simulink model "HLF_SystemArchitecture"  (R2024a)
settings: Solver=VariableStepAuto  StartTime=0.0  StopTime=10.0  RelTol=1e-3
undefined symbols (not defined in the file): Deceleration, LIN_Acceleration
settings Model: DataDictionary=DD_HLF_DataTypes.sldd  Creator=The MathWorks, Inc.  LastModifiedBy=The MathWorks, Inc.
settings SolverCC: AlgebraicLoopSolver=TrustRegion  MaxZcPerStep=1
settings DebuggingCC: UnconnectedInputMsg=warning  UnconnectedOutputMsg=warning  UnconnectedLineMsg=warning
settings ModelReferenceCC: EnableRefExpFcnMdlSchedulingChecks=on
settings RTWCC: GPUComputeCapability=3.5  DLArmComputeVersion=19.05

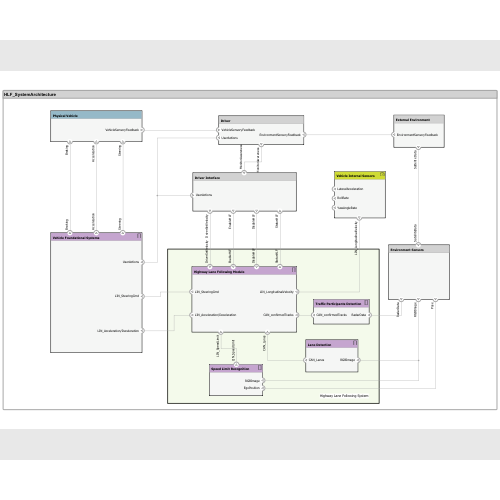
[thumbnail: Simulink's stored preview of the top-level diagram]
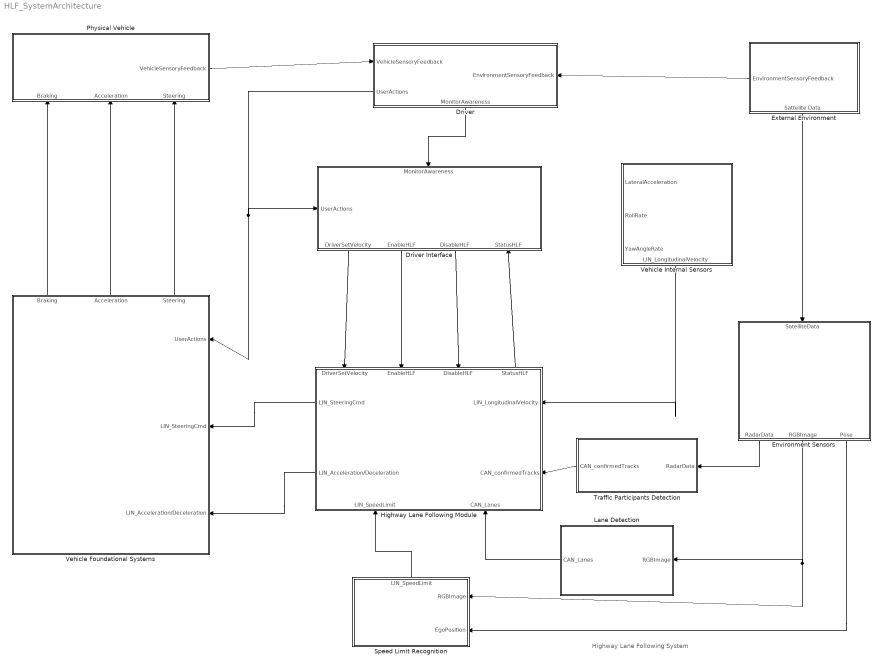
== system HLF_SystemArchitecture ==
  note: Highway Lane Following System
  Driver : Subsystem
      settings: PortSchema="{\"entries\":[{\"content\":{\"headerSize\":26,\"margin\":15,\"minimumSpacing\":25,\"sides\":[{\"content\":{\"connectorIds\":[\"In1\",\"Out2\"]},\"type\":\"ConnectorPlacement.EquallySpacedRectSide\",\"uuid\":\"57d9105b-5891-4b67-8053-94876359dbfc\"},{\"content\":{\"connectorIds\":[\"In2\"],\"side\":\"RIGHT\"},\"type\":\"ConnectorPlacement.EquallySpacedRectSide\",\"uuid\":\"3fd4430d-d88a-4c36-b7db-738c17ba6bd1\"},{\"content\":{\"connectorIds\":[],\"side\":\"TOP\"},\"type\":\"ConnectorPlacement.EquallySpacedRectSide\",\"uuid\":\"61a8faa4-d042-4724-a03b-b771d37b6fdb\"},{\"content\":{\"connectorIds\":[\"Out1\"],\"side\":\"BOTTOM\"},\"type\":\"ConnectorPlacement.EquallySpacedRectSide\",\"uuid\":\"67674867-d4fb-4781-a637-daf086112980\"},{\"content\":{\"connectorIds\":[],\"side\":\"HIDDEN\"},\"type\":\"ConnectorPlacement.EquallySpacedRectSide\",\"uuid\":\"dc3c6b25-4da2-48ee-a238-2c1d12fb30ea\"}]},\"type\":\"ConnectorPlacement.EquallySpacedConnector\",\"uuid\":\"fbcd43a8-976e-4463-97d1-0d40c2a22b40\"}],\"packageUris\":[\"http://schema.mathworks.com/mf0/Connector/R2020b\"],\"version\":\"1.0\"}"
  Driver Interface : Subsystem
      settings: PortSchema="{\"entries\":[{\"content\":{\"headerSize\":26,\"margin\":15,\"minimumSpacing\":25,\"sides\":[{\"content\":{\"connectorIds\":[\"In3\"]},\"type\":\"ConnectorPlacement.EquallySpacedRectSide\",\"uuid\":\"b5c560bf-b1de-4f7d-bfcc-f34083c77ac8\"},{\"content\":{\"connectorIds\":[],\"side\":\"RIGHT\"},\"type\":\"ConnectorPlacement.EquallySpacedRectSide\",\"uuid\":\"ae8c8d4f-55e3-4192-b0d3-7950d45edb35\"},{\"content\":{\"connectorIds\":[\"In2\"],\"side\":\"TOP\"},\"type\":\"ConnectorPlacement.EquallySpacedRectSide\",\"uuid\":\"be988242-c8a1-4b97-b048-993c7975a175\"},{\"content\":{\"connectorIds\":[\"Out1\",\"Out2\",\"Out3\",\"In1\"],\"side\":\"BOTTOM\"},\"type\":\"ConnectorPlacement.EquallySpacedRectSide\",\"uuid\":\"b880dce2-1370-4b6b-af53-719174202621\"},{\"content\":{\"connectorIds\":[],\"side\":\"HIDDEN\"},\"type\":\"ConnectorPlacement.EquallySpacedRectSide\",\"uuid\":\"95e462f2-ec2c-4474-9ace-7d27c2e08c82\"}]},\"type\":\"ConnectorPlacement.EquallySpacedConnector\",\"uuid\":\"71deff37-1671-43b5-b896-1963241a26e4\"}],\"packageUris\":[\"http://schema.mathworks.com/mf0/Connector/R2020b\"],\"version\":\"1.0\"}"
  Environment Sensors : Subsystem
      settings: PortSchema="{\"entries\":[{\"content\":{\"headerSize\":26,\"margin\":15,\"minimumSpacing\":25,\"sides\":[{\"content\":{\"connectorIds\":[]},\"type\":\"ConnectorPlacement.EquallySpacedRectSide\",\"uuid\":\"57d9105b-5891-4b67-8053-94876359dbfc\"},{\"content\":{\"connectorIds\":[],\"side\":\"RIGHT\"},\"type\":\"ConnectorPlacement.EquallySpacedRectSide\",\"uuid\":\"3fd4430d-d88a-4c36-b7db-738c17ba6bd1\"},{\"content\":{\"connectorIds\":[\"In1\"],\"side\":\"TOP\"},\"type\":\"ConnectorPlacement.EquallySpacedRectSide\",\"uuid\":\"61a8faa4-d042-4724-a03b-b771d37b6fdb\"},{\"content\":{\"connectorIds\":[\"Out2\",\"Out1\",\"Out3\"],\"side\":\"BOTTOM\"},\"type\":\"ConnectorPlacement.EquallySpacedRectSide\",\"uuid\":\"235332e3-de05-4da1-8ee5-464085e16b9c\"},{\"content\":{\"connectorIds\":[],\"side\":\"HIDDEN\"},\"type\":\"ConnectorPlacement.EquallySpacedRectSide\",\"uuid\":\"dc3c6b25-4da2-48ee-a238-2c1d12fb30ea\"}]},\"type\":\"ConnectorPlacement.EquallySpacedConnector\",\"uuid\":\"fbcd43a8-976e-4463-97d1-0d40c2a22b40\"}],\"packageUris\":[\"http://schema.mathworks.com/mf0/Connector/R2020b\"],\"version\":\"1.0\"}"
  External Environment : Subsystem
      settings: PortSchema="{\"entries\":[{\"content\":{\"headerSize\":26,\"margin\":15,\"minimumSpacing\":25,\"sides\":[{\"content\":{\"connectorIds\":[\"Out1\"]},\"type\":\"ConnectorPlacement.EquallySpacedRectSide\",\"uuid\":\"57d9105b-5891-4b67-8053-94876359dbfc\"},{\"content\":{\"connectorIds\":[],\"side\":\"RIGHT\"},\"type\":\"ConnectorPlacement.EquallySpacedRectSide\",\"uuid\":\"3fd4430d-d88a-4c36-b7db-738c17ba6bd1\"},{\"content\":{\"connectorIds\":[],\"side\":\"TOP\"},\"type\":\"ConnectorPlacement.EquallySpacedRectSide\",\"uuid\":\"61a8faa4-d042-4724-a03b-b771d37b6fdb\"},{\"content\":{\"connectorIds\":[\"Out2\"],\"side\":\"BOTTOM\"},\"type\":\"ConnectorPlacement.EquallySpacedRectSide\",\"uuid\":\"9a94a6b5-3a5b-4073-ae25-fdf18980dc03\"},{\"content\":{\"connectorIds\":[],\"side\":\"HIDDEN\"},\"type\":\"ConnectorPlacement.EquallySpacedRectSide\",\"uuid\":\"dc3c6b25-4da2-48ee-a238-2c1d12fb30ea\"}]},\"type\":\"ConnectorPlacement.EquallySpacedConnector\",\"uuid\":\"fbcd43a8-976e-4463-97d1-0d40c2a22b40\"}],\"packageUris\":[\"http://schema.mathworks.com/mf0/Connector/R2020b\"],\"version\":\"1.0\"}"
  Highway Lane Following Module : Subsystem
      settings: PortSchema="{\"entries\":[{\"content\":{\"headerSize\":26,\"margin\":15,\"minimumSpacing\":25,\"sides\":[{\"content\":{\"connectorIds\":[\"Out1\",\"Out2\"]},\"type\":\"ConnectorPlacement.EquallySpacedRectSide\",\"uuid\":\"5982ae23-38c5-467f-966f-0de5138e6d7a\"},{\"content\":{\"connectorIds\":[\"In6\",\"In7\"],\"side\":\"RIGHT\"},\"type\":\"ConnectorPlacement.EquallySpacedRectSide\",\"uuid\":\"84362337-a9b7-4030-aff8-83ed548d578d\"},{\"content\":{\"connectorIds\":[\"In2\",\"In3\",\"In4\",\"Out3\"],\"side\":\"TOP\"},\"type\":\"ConnectorPlacement.EquallySpacedRectSide\",\"uuid\":\"856fe994-3ca2-486c-b816-04bdae2310a8\"},{\"content\":{\"connectorIds\":[\"In1\",\"In5\"],\"side\":\"BOTTOM\"},\"type\":\"ConnectorPlacement.EquallySpacedRectSide\",\"uuid\":\"0d12cb15-66d1-47ae-a3bb-95c751ef0d09\"}]},\"type\":\"ConnectorPlacement.EquallySpacedConnector\",\"uuid\":\"ebc65c4e-e942-490a-8c6c-35e3db9f64d6\"}],\"packageUris\":[\"http://schema.mathworks.com/mf0/Connector/R2020b\"],\"version\":\"1.0\"}"
  Lane Detection : Subsystem
      settings: PortSchema="{\"entries\":[{\"content\":{\"headerSize\":26,\"margin\":15,\"minimumSpacing\":25,\"sides\":[{\"content\":{\"connectorIds\":[\"Out1\"]},\"type\":\"ConnectorPlacement.EquallySpacedRectSide\",\"uuid\":\"b5c560bf-b1de-4f7d-bfcc-f34083c77ac8\"},{\"content\":{\"connectorIds\":[\"In1\"],\"side\":\"RIGHT\"},\"type\":\"ConnectorPlacement.EquallySpacedRectSide\",\"uuid\":\"ae8c8d4f-55e3-4192-b0d3-7950d45edb35\"},{\"content\":{\"connectorIds\":[],\"side\":\"TOP\"},\"type\":\"ConnectorPlacement.EquallySpacedRectSide\",\"uuid\":\"be988242-c8a1-4b97-b048-993c7975a175\"},{\"content\":{\"connectorIds\":[],\"side\":\"HIDDEN\"},\"type\":\"ConnectorPlacement.EquallySpacedRectSide\",\"uuid\":\"95e462f2-ec2c-4474-9ace-7d27c2e08c82\"}]},\"type\":\"ConnectorPlacement.EquallySpacedConnector\",\"uuid\":\"71deff37-1671-43b5-b896-1963241a26e4\"}],\"packageUris\":[\"http://schema.mathworks.com/mf0/Connector/R2020b\"],\"version\":\"1.0\"}"
  Physical Vehicle : Subsystem
      settings: PortSchema="{\"entries\":[{\"content\":{\"headerSize\":26,\"margin\":15,\"minimumSpacing\":25,\"sides\":[{\"content\":{\"connectorIds\":[]},\"type\":\"ConnectorPlacement.EquallySpacedRectSide\",\"uuid\":\"57d9105b-5891-4b67-8053-94876359dbfc\"},{\"content\":{\"connectorIds\":[\"Out1\"],\"side\":\"RIGHT\"},\"type\":\"ConnectorPlacement.EquallySpacedRectSide\",\"uuid\":\"3fd4430d-d88a-4c36-b7db-738c17ba6bd1\"},{\"content\":{\"connectorIds\":[],\"side\":\"TOP\"},\"type\":\"ConnectorPlacement.EquallySpacedRectSide\",\"uuid\":\"61a8faa4-d042-4724-a03b-b771d37b6fdb\"},{\"content\":{\"connectorIds\":[\"In1\",\"In2\",\"In3\"],\"side\":\"BOTTOM\"},\"type\":\"ConnectorPlacement.EquallySpacedRectSide\",\"uuid\":\"80043eee-7869-4f7b-9f18-53002ef55b49\"},{\"content\":{\"connectorIds\":[],\"side\":\"HIDDEN\"},\"type\":\"ConnectorPlacement.EquallySpacedRectSide\",\"uuid\":\"dc3c6b25-4da2-48ee-a238-2c1d12fb30ea\"}]},\"type\":\"ConnectorPlacement.EquallySpacedConnector\",\"uuid\":\"fbcd43a8-976e-4463-97d1-0d40c2a22b40\"}],\"packageUris\":[\"http://schema.mathworks.com/mf0/Connector/R2020b\"],\"version\":\"1.0\"}"
  Speed Limit Recognition : Subsystem
      settings: PortSchema="{\"entries\":[{\"content\":{\"headerSize\":26,\"margin\":15,\"minimumSpacing\":25,\"sides\":[{\"content\":{\"connectorIds\":[]},\"type\":\"ConnectorPlacement.EquallySpacedRectSide\",\"uuid\":\"b5c560bf-b1de-4f7d-bfcc-f34083c77ac8\"},{\"content\":{\"connectorIds\":[\"In1\",\"In2\"],\"side\":\"RIGHT\"},\"type\":\"ConnectorPlacement.EquallySpacedRectSide\",\"uuid\":\"ae8c8d4f-55e3-4192-b0d3-7950d45edb35\"},{\"content\":{\"connectorIds\":[\"Out1\"],\"side\":\"TOP\"},\"type\":\"ConnectorPlacement.EquallySpacedRectSide\",\"uuid\":\"be988242-c8a1-4b97-b048-993c7975a175\"},{\"content\":{\"connectorIds\":[],\"side\":\"HIDDEN\"},\"type\":\"ConnectorPlacement.EquallySpacedRectSide\",\"uuid\":\"95e462f2-ec2c-4474-9ace-7d27c2e08c82\"}]},\"type\":\"ConnectorPlacement.EquallySpacedConnector\",\"uuid\":\"71deff37-1671-43b5-b896-1963241a26e4\"}],\"packageUris\":[\"http://schema.mathworks.com/mf0/Connector/R2020b\"],\"version\":\"1.0\"}"
  Traffic Participants Detection : Subsystem
      settings: PortSchema="{\"entries\":[{\"content\":{\"headerSize\":26,\"margin\":15,\"minimumSpacing\":25,\"sides\":[{\"content\":{\"connectorIds\":[\"Out1\"]},\"type\":\"ConnectorPlacement.EquallySpacedRectSide\",\"uuid\":\"b5c560bf-b1de-4f7d-bfcc-f34083c77ac8\"},{\"content\":{\"connectorIds\":[\"In1\"],\"side\":\"RIGHT\"},\"type\":\"ConnectorPlacement.EquallySpacedRectSide\",\"uuid\":\"ae8c8d4f-55e3-4192-b0d3-7950d45edb35\"},{\"content\":{\"connectorIds\":[],\"side\":\"TOP\"},\"type\":\"ConnectorPlacement.EquallySpacedRectSide\",\"uuid\":\"be988242-c8a1-4b97-b048-993c7975a175\"},{\"content\":{\"connectorIds\":[],\"side\":\"HIDDEN\"},\"type\":\"ConnectorPlacement.EquallySpacedRectSide\",\"uuid\":\"95e462f2-ec2c-4474-9ace-7d27c2e08c82\"}]},\"type\":\"ConnectorPlacement.EquallySpacedConnector\",\"uuid\":\"71deff37-1671-43b5-b896-1963241a26e4\"}],\"packageUris\":[\"http://schema.mathworks.com/mf0/Connector/R2020b\"],\"version\":\"1.0\"}"
  Vehicle Foundational Systems : Subsystem
      settings: PortSchema="{\"entries\":[{\"content\":{\"headerSize\":26,\"margin\":15,\"minimumSpacing\":25,\"sides\":[{\"content\":{\"connectorIds\":[]},\"type\":\"ConnectorPlacement.EquallySpacedRectSide\",\"uuid\":\"b5c560bf-b1de-4f7d-bfcc-f34083c77ac8\"},{\"content\":{\"connectorIds\":[\"In1\",\"In2\",\"In3\"],\"side\":\"RIGHT\"},\"type\":\"ConnectorPlacement.EquallySpacedRectSide\",\"uuid\":\"ae8c8d4f-55e3-4192-b0d3-7950d45edb35\"},{\"content\":{\"connectorIds\":[\"Out1\",\"Out2\",\"Out3\"],\"side\":\"TOP\"},\"type\":\"ConnectorPlacement.EquallySpacedRectSide\",\"uuid\":\"be988242-c8a1-4b97-b048-993c7975a175\"},{\"content\":{\"connectorIds\":[],\"side\":\"HIDDEN\"},\"type\":\"ConnectorPlacement.EquallySpacedRectSide\",\"uuid\":\"95e462f2-ec2c-4474-9ace-7d27c2e08c82\"}]},\"type\":\"ConnectorPlacement.EquallySpacedConnector\",\"uuid\":\"71deff37-1671-43b5-b896-1963241a26e4\"}],\"packageUris\":[\"http://schema.mathworks.com/mf0/Connector/R2020b\"],\"version\":\"1.0\"}"
  Vehicle Internal Sensors : Subsystem
      settings: PortSchema="{\"entries\":[{\"content\":{\"headerSize\":26,\"margin\":15,\"minimumSpacing\":25,\"sides\":[{\"content\":{\"connectorIds\":[\"Out1\",\"Out2\",\"Out3\"]},\"type\":\"ConnectorPlacement.EquallySpacedRectSide\",\"uuid\":\"57d9105b-5891-4b67-8053-94876359dbfc\"},{\"content\":{\"connectorIds\":[],\"side\":\"RIGHT\"},\"type\":\"ConnectorPlacement.EquallySpacedRectSide\",\"uuid\":\"3fd4430d-d88a-4c36-b7db-738c17ba6bd1\"},{\"content\":{\"connectorIds\":[],\"side\":\"TOP\"},\"type\":\"ConnectorPlacement.EquallySpacedRectSide\",\"uuid\":\"61a8faa4-d042-4724-a03b-b771d37b6fdb\"},{\"content\":{\"connectorIds\":[\"Out4\"],\"side\":\"BOTTOM\"},\"type\":\"ConnectorPlacement.EquallySpacedRectSide\",\"uuid\":\"df0d5577-7196-4d99-9ad6-c722a9507efd\"},{\"content\":{\"connectorIds\":[],\"side\":\"HIDDEN\"},\"type\":\"ConnectorPlacement.EquallySpacedRectSide\",\"uuid\":\"dc3c6b25-4da2-48ee-a238-2c1d12fb30ea\"}]},\"type\":\"ConnectorPlacement.EquallySpacedConnector\",\"uuid\":\"fbcd43a8-976e-4463-97d1-0d40c2a22b40\"}],\"packageUris\":[\"http://schema.mathworks.com/mf0/Connector/R2020b\"],\"version\":\"1.0\"}"
  wires:
  External Environment/2(Sattelite Data) -> Environment Sensors/1(SatelliteData)
  Driver/1(MonitorAwareness) -> Driver Interface/2(MonitorAwareness)
  Driver/2(UserActions) -> Vehicle Foundational Systems/1(UserActions), Driver Interface/3(UserActions)
  External Environment/1(EnvironmentSensoryFeedback) -> Driver/2(EnvironmentSensoryFeedback)
  Environment Sensors/2(RadarData) -> Traffic Participants Detection/1(RadarData)
  Traffic Participants Detection/1(CAN_confirmedTracks) -> Highway Lane Following Module/7(CAN_confirmedTracks)
  Lane Detection/1(CAN_Lanes) -> Highway Lane Following Module/5(CAN_Lanes)
  Environment Sensors/1(RGBImage) -> Speed Limit Recognition/1(RGBImage), Lane Detection/1(RGBImage)
  Speed Limit Recognition/1(LIN_SpeedLimit) -> Highway Lane Following Module/1(LIN_SpeedLimit)
  Vehicle Foundational Systems/3(Steering) -> Physical Vehicle/3(Steering)
  Vehicle Foundational Systems/2(Acceleration) -> Physical Vehicle/2(Acceleration)
  Vehicle Foundational Systems/1(Braking) -> Physical Vehicle/1(Braking)
  Highway Lane Following Module/1(LIN_SteeringCmd) -> Vehicle Foundational Systems/2(LIN_SteeringCmd)
  Highway Lane Following Module/2(LIN_Acceleration/Deceleration) -> Vehicle Foundational Systems/3(LIN_Acceleration/Deceleration)
  Driver Interface/2(EnableHLF) -> Highway Lane Following Module/3(EnableHLF)
  Environment Sensors/3(Pose) -> Speed Limit Recognition/2(EgoPosition)
  Driver Interface/1(DriverSetVelocity) -> Highway Lane Following Module/2(DriverSetVelocity)
  Driver Interface/3(DisableHLF) -> Highway Lane Following Module/4(DisableHLF)
  Highway Lane Following Module/3(StatusHLF) -> Driver Interface/1(StatusHLF)
  Vehicle Internal Sensors/4(LIN_LongitudinalVelocity) -> Highway Lane Following Module/6(LIN_LongitudinalVelocity)
  Physical Vehicle/1(VehicleSensoryFeedback) -> Driver/1(VehicleSensoryFeedback)

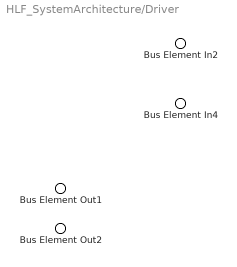
== system HLF_SystemArchitecture/Driver ==
  Bus Element In2 : Inport  PortName=VehicleSensoryFeedback
  Bus Element In4 : Inport  Port=2  PortName=EnvironmentSensoryFeedback
  Bus Element Out1 : Outport  PortName=MonitorAwareness
  Bus Element Out2 : Outport  Port=2  PortName=UserActions

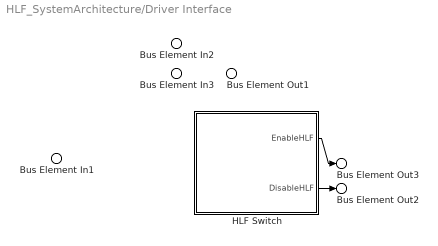
== system HLF_SystemArchitecture/Driver Interface ==
  Bus Element In3 : Inport  PortName=StatusHLF
  Bus Element In2 : Inport  Port=2  PortName=MonitorAwareness
  Bus Element In1 : Inport  Port=3  PortName=UserActions
  HLF Switch : Subsystem
      settings: PortSchema="{\"entries\":[{\"content\":{\"headerSize\":26,\"margin\":15,\"minimumSpacing\":25,\"sides\":[{\"content\":{\"connectorIds\":[]},\"type\":\"ConnectorPlacement.EquallySpacedRectSide\",\"uuid\":\"b7f407b7-33e8-47f4-a6de-9d0843597b8d\"},{\"content\":{\"connectorIds\":[\"Out1\",\"Out2\"],\"side\":\"RIGHT\"},\"type\":\"ConnectorPlacement.EquallySpacedRectSide\",\"uuid\":\"c67fba66-c883-4563-bb96-6929606b6eb1\"},{\"content\":{\"connectorIds\":[],\"side\":\"TOP\"},\"type\":\"ConnectorPlacement.EquallySpacedRectSide\",\"uuid\":\"b02a73e2-c76f-4a23-855b-ce43e445bb81\"}]},\"type\":\"ConnectorPlacement.EquallySpacedConnector\",\"uuid\":\"68a829ea-ceae-4477-bf03-0573732a373e\"}],\"packageUris\":[\"http://schema.mathworks.com/mf0/Connector/R2020b\"],\"version\":\"1.0\"}"
  Bus Element Out1 : Outport  PortName=DriverSetVelocity
  Bus Element Out3 : Outport  Port=2  PortName=EnableHLF
  Bus Element Out2 : Outport  Port=3  PortName=DisableHLF
  wires:
  HLF Switch/1(EnableHLF) -> Bus Element Out3/1
  HLF Switch/2(DisableHLF) -> Bus Element Out2/1

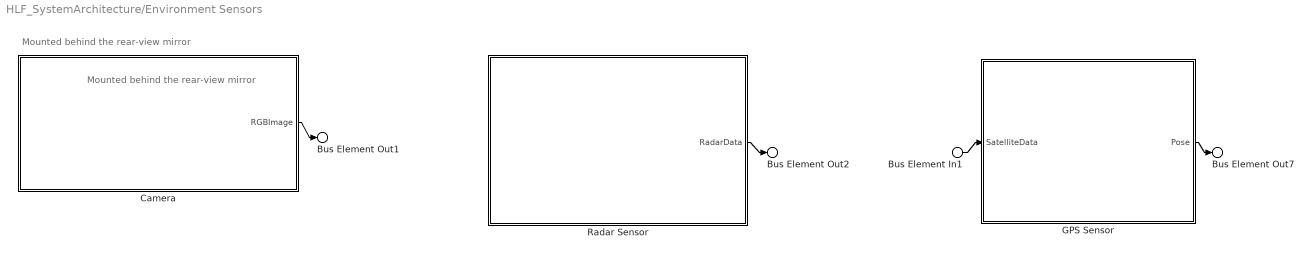
== system HLF_SystemArchitecture/Environment Sensors ==
  note: Mounted behind the rear-view mirror
  note: Mounted behind the rear-view mirror
  Bus Element In1 : Inport  PortName=SatelliteData
  "Camera " : Subsystem
      settings: PortSchema="{\"entries\":[{\"content\":{\"headerSize\":26,\"margin\":15,\"minimumSpacing\":25,\"sides\":[{\"content\":{\"connectorIds\":[]},\"type\":\"ConnectorPlacement.EquallySpacedRectSide\",\"uuid\":\"57d9105b-5891-4b67-8053-94876359dbfc\"},{\"content\":{\"connectorIds\":[\"Out1\"],\"side\":\"RIGHT\"},\"type\":\"ConnectorPlacement.EquallySpacedRectSide\",\"uuid\":\"3fd4430d-d88a-4c36-b7db-738c17ba6bd1\"},{\"content\":{\"connectorIds\":[],\"side\":\"TOP\"},\"type\":\"ConnectorPlacement.EquallySpacedRectSide\",\"uuid\":\"61a8faa4-d042-4724-a03b-b771d37b6fdb\"},{\"content\":{\"connectorIds\":[],\"side\":\"BOTTOM\"},\"type\":\"ConnectorPlacement.EquallySpacedRectSide\",\"uuid\":\"084da6be-2921-4dfe-a8dc-b8025c48e485\"},{\"content\":{\"connectorIds\":[],\"side\":\"HIDDEN\"},\"type\":\"ConnectorPlacement.EquallySpacedRectSide\",\"uuid\":\"dc3c6b25-4da2-48ee-a238-2c1d12fb30ea\"}]},\"type\":\"ConnectorPlacement.EquallySpacedConnector\",\"uuid\":\"fbcd43a8-976e-4463-97d1-0d40c2a22b40\"}],\"packageUris\":[\"http://schema.mathworks.com/mf0/Connector/R2020b\"],\"version\":\"1.0\"}"
  GPS Sensor : Subsystem
      settings: PortSchema="{\"entries\":[{\"content\":{\"headerSize\":26,\"margin\":15,\"minimumSpacing\":25,\"sides\":[{\"content\":{\"connectorIds\":[\"In1\"]},\"type\":\"ConnectorPlacement.EquallySpacedRectSide\",\"uuid\":\"b5c560bf-b1de-4f7d-bfcc-f34083c77ac8\"},{\"content\":{\"connectorIds\":[\"Out1\"],\"side\":\"RIGHT\"},\"type\":\"ConnectorPlacement.EquallySpacedRectSide\",\"uuid\":\"ae8c8d4f-55e3-4192-b0d3-7950d45edb35\"},{\"content\":{\"connectorIds\":[],\"side\":\"TOP\"},\"type\":\"ConnectorPlacement.EquallySpacedRectSide\",\"uuid\":\"be988242-c8a1-4b97-b048-993c7975a175\"},{\"content\":{\"connectorIds\":[],\"side\":\"HIDDEN\"},\"type\":\"ConnectorPlacement.EquallySpacedRectSide\",\"uuid\":\"95e462f2-ec2c-4474-9ace-7d27c2e08c82\"}]},\"type\":\"ConnectorPlacement.EquallySpacedConnector\",\"uuid\":\"71deff37-1671-43b5-b896-1963241a26e4\"}],\"packageUris\":[\"http://schema.mathworks.com/mf0/Connector/R2020b\"],\"version\":\"1.0\"}"
  Radar Sensor : Subsystem
      settings: PortSchema="{\"entries\":[{\"content\":{\"headerSize\":26,\"margin\":15,\"minimumSpacing\":25,\"sides\":[{\"content\":{\"connectorIds\":[]},\"type\":\"ConnectorPlacement.EquallySpacedRectSide\",\"uuid\":\"57d9105b-5891-4b67-8053-94876359dbfc\"},{\"content\":{\"connectorIds\":[\"Out1\"],\"side\":\"RIGHT\"},\"type\":\"ConnectorPlacement.EquallySpacedRectSide\",\"uuid\":\"3fd4430d-d88a-4c36-b7db-738c17ba6bd1\"},{\"content\":{\"connectorIds\":[],\"side\":\"TOP\"},\"type\":\"ConnectorPlacement.EquallySpacedRectSide\",\"uuid\":\"61a8faa4-d042-4724-a03b-b771d37b6fdb\"},{\"content\":{\"connectorIds\":[],\"side\":\"HIDDEN\"},\"type\":\"ConnectorPlacement.EquallySpacedRectSide\",\"uuid\":\"dc3c6b25-4da2-48ee-a238-2c1d12fb30ea\"}]},\"type\":\"ConnectorPlacement.EquallySpacedConnector\",\"uuid\":\"fbcd43a8-976e-4463-97d1-0d40c2a22b40\"}],\"packageUris\":[\"http://schema.mathworks.com/mf0/Connector/R2020b\"],\"version\":\"1.0\"}"
  Bus Element Out1 : Outport  PortName=RGBImage
  Bus Element Out2 : Outport  Port=2  PortName=RadarData
  Bus Element Out7 : Outport  Port=3  PortName=Pose
  wires:
  "Camera "/1(RGBImage) -> Bus Element Out1/1
  Radar Sensor/1(RadarData) -> Bus Element Out2/1
  Bus Element In1/1 -> GPS Sensor/1(SatelliteData)
  GPS Sensor/1(Pose) -> Bus Element Out7/1

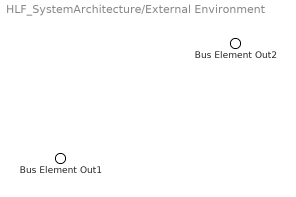
== system HLF_SystemArchitecture/External Environment ==
  Bus Element Out2 : Outport  PortName=EnvironmentSensoryFeedback
  Bus Element Out1 : Outport  Port=2  PortName=Sattelite Data

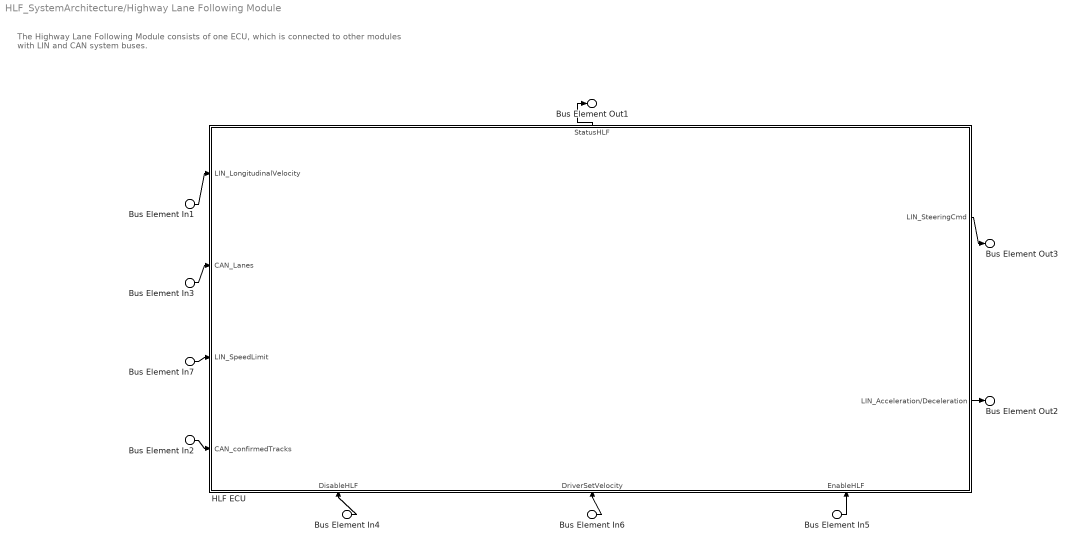
== system HLF_SystemArchitecture/Highway Lane Following Module ==
  note: The Highway Lane Following Module consists of one ECU, which is connected to other modules with LIN and CAN system buses.
  Bus Element In7 : Inport  PortName=LIN_SpeedLimit
  Bus Element In6 : Inport  Port=2  PortName=DriverSetVelocity
  Bus Element In5 : Inport  Port=3  PortName=EnableHLF
  Bus Element In4 : Inport  Port=4  PortName=DisableHLF
  Bus Element In3 : Inport  Port=5  PortName=CAN_Lanes
  Bus Element In1 : Inport  Port=6  PortName=LIN_LongitudinalVelocity
  Bus Element In2 : Inport  Port=7  PortName=CAN_confirmedTracks
  HLF ECU : Subsystem
      settings: PortSchema="{\"entries\":[{\"content\":{\"headerSize\":26,\"margin\":15,\"minimumSpacing\":25,\"sides\":[{\"content\":{\"connectorIds\":[\"In4\",\"In7\",\"In6\",\"In5\"]},\"type\":\"ConnectorPlacement.EquallySpacedRectSide\",\"uuid\":\"5982ae23-38c5-467f-966f-0de5138e6d7a\"},{\"content\":{\"connectorIds\":[\"Out1\",\"Out2\"],\"side\":\"RIGHT\"},\"type\":\"ConnectorPlacement.EquallySpacedRectSide\",\"uuid\":\"84362337-a9b7-4030-aff8-83ed548d578d\"},{\"content\":{\"connectorIds\":[\"Out3\"],\"side\":\"TOP\"},\"type\":\"ConnectorPlacement.EquallySpacedRectSide\",\"uuid\":\"856fe994-3ca2-486c-b816-04bdae2310a8\"},{\"content\":{\"connectorIds\":[\"In2\",\"In3\",\"In1\"],\"side\":\"BOTTOM\"},\"type\":\"ConnectorPlacement.EquallySpacedRectSide\",\"uuid\":\"42e90607-69cd-4d6c-8280-b0cc067697ba\"}]},\"type\":\"ConnectorPlacement.EquallySpacedConnector\",\"uuid\":\"ebc65c4e-e942-490a-8c6c-35e3db9f64d6\"}],\"packageUris\":[\"http://schema.mathworks.com/mf0/Connector/R2020b\"],\"version\":\"1.0\"}"
  Bus Element Out3 : Outport  PortName=LIN_SteeringCmd
  Bus Element Out2 : Outport  Port=2  PortName=LIN_Acceleration/Deceleration
  Bus Element Out1 : Outport  Port=3  PortName=StatusHLF
  wires:
  Bus Element In7/1 -> HLF ECU/6(LIN_SpeedLimit)
  Bus Element In3/1 -> HLF ECU/7(CAN_Lanes)
  HLF ECU/1(LIN_SteeringCmd) -> Bus Element Out3/1
  HLF ECU/2(LIN_Acceleration/Deceleration) -> Bus Element Out2/1
  Bus Element In1/1 -> HLF ECU/4(LIN_LongitudinalVelocity)
  Bus Element In2/1 -> HLF ECU/5(CAN_confirmedTracks)
  Bus Element In6/1 -> HLF ECU/3(DriverSetVelocity)
  Bus Element In5/1 -> HLF ECU/1(EnableHLF)
  Bus Element In4/1 -> HLF ECU/2(DisableHLF)
  HLF ECU/3(StatusHLF) -> Bus Element Out1/1

== system HLF_SystemArchitecture/Lane Detection ==
  Bus Element In1 : Inport  PortName=RGBImage
  Bus Element Out1 : Outport  PortName=CAN_Lanes

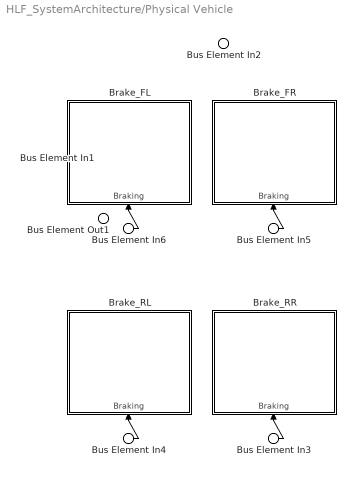
== system HLF_SystemArchitecture/Physical Vehicle ==
  Bus Element In{3..6} (4 alike) : Inport  PortName=Braking
  Bus Element In2 : Inport  Port=2  PortName=Acceleration
  Bus Element In1 : Inport  Port=3  PortName=Steering
  Brake_FL : Subsystem
      settings: PortSchema="{\"entries\":[{\"content\":{\"headerSize\":26,\"margin\":15,\"minimumSpacing\":25,\"sides\":[{\"content\":{\"connectorIds\":[]},\"type\":\"ConnectorPlacement.EquallySpacedRectSide\",\"uuid\":\"b7f407b7-33e8-47f4-a6de-9d0843597b8d\"},{\"content\":{\"connectorIds\":[],\"side\":\"RIGHT\"},\"type\":\"ConnectorPlacement.EquallySpacedRectSide\",\"uuid\":\"c67fba66-c883-4563-bb96-6929606b6eb1\"},{\"content\":{\"connectorIds\":[],\"side\":\"TOP\"},\"type\":\"ConnectorPlacement.EquallySpacedRectSide\",\"uuid\":\"b02a73e2-c76f-4a23-855b-ce43e445bb81\"},{\"content\":{\"connectorIds\":[\"In1\"],\"side\":\"BOTTOM\"},\"type\":\"ConnectorPlacement.EquallySpacedRectSide\",\"uuid\":\"2822b3d2-5412-4a59-b682-69e362d996e9\"}]},\"type\":\"ConnectorPlacement.EquallySpacedConnector\",\"uuid\":\"68a829ea-ceae-4477-bf03-0573732a373e\"}],\"packageUris\":[\"http://schema.mathworks.com/mf0/Connector/R2020b\"],\"version\":\"1.0\"}"
  Brake_FR : Subsystem
      settings: PortSchema="{\"entries\":[{\"content\":{\"headerSize\":26,\"margin\":15,\"minimumSpacing\":25,\"sides\":[{\"content\":{\"connectorIds\":[]},\"type\":\"ConnectorPlacement.EquallySpacedRectSide\",\"uuid\":\"b7f407b7-33e8-47f4-a6de-9d0843597b8d\"},{\"content\":{\"connectorIds\":[],\"side\":\"RIGHT\"},\"type\":\"ConnectorPlacement.EquallySpacedRectSide\",\"uuid\":\"c67fba66-c883-4563-bb96-6929606b6eb1\"},{\"content\":{\"connectorIds\":[],\"side\":\"TOP\"},\"type\":\"ConnectorPlacement.EquallySpacedRectSide\",\"uuid\":\"b02a73e2-c76f-4a23-855b-ce43e445bb81\"},{\"content\":{\"connectorIds\":[\"In1\"],\"side\":\"BOTTOM\"},\"type\":\"ConnectorPlacement.EquallySpacedRectSide\",\"uuid\":\"f55a7542-8702-4f3b-9ddf-b68a959d2755\"}]},\"type\":\"ConnectorPlacement.EquallySpacedConnector\",\"uuid\":\"68a829ea-ceae-4477-bf03-0573732a373e\"}],\"packageUris\":[\"http://schema.mathworks.com/mf0/Connector/R2020b\"],\"version\":\"1.0\"}"
  Brake_RL : Subsystem
      settings: PortSchema="{\"entries\":[{\"content\":{\"headerSize\":26,\"margin\":15,\"minimumSpacing\":25,\"sides\":[{\"content\":{\"connectorIds\":[]},\"type\":\"ConnectorPlacement.EquallySpacedRectSide\",\"uuid\":\"b7f407b7-33e8-47f4-a6de-9d0843597b8d\"},{\"content\":{\"connectorIds\":[],\"side\":\"RIGHT\"},\"type\":\"ConnectorPlacement.EquallySpacedRectSide\",\"uuid\":\"c67fba66-c883-4563-bb96-6929606b6eb1\"},{\"content\":{\"connectorIds\":[],\"side\":\"TOP\"},\"type\":\"ConnectorPlacement.EquallySpacedRectSide\",\"uuid\":\"b02a73e2-c76f-4a23-855b-ce43e445bb81\"},{\"content\":{\"connectorIds\":[\"In1\"],\"side\":\"BOTTOM\"},\"type\":\"ConnectorPlacement.EquallySpacedRectSide\",\"uuid\":\"16d69be7-3f1c-40af-bb9c-59d3923159c6\"}]},\"type\":\"ConnectorPlacement.EquallySpacedConnector\",\"uuid\":\"68a829ea-ceae-4477-bf03-0573732a373e\"}],\"packageUris\":[\"http://schema.mathworks.com/mf0/Connector/R2020b\"],\"version\":\"1.0\"}"
  Brake_RR : Subsystem
      settings: PortSchema="{\"entries\":[{\"content\":{\"headerSize\":26,\"margin\":15,\"minimumSpacing\":25,\"sides\":[{\"content\":{\"connectorIds\":[]},\"type\":\"ConnectorPlacement.EquallySpacedRectSide\",\"uuid\":\"b7f407b7-33e8-47f4-a6de-9d0843597b8d\"},{\"content\":{\"connectorIds\":[],\"side\":\"RIGHT\"},\"type\":\"ConnectorPlacement.EquallySpacedRectSide\",\"uuid\":\"c67fba66-c883-4563-bb96-6929606b6eb1\"},{\"content\":{\"connectorIds\":[],\"side\":\"TOP\"},\"type\":\"ConnectorPlacement.EquallySpacedRectSide\",\"uuid\":\"b02a73e2-c76f-4a23-855b-ce43e445bb81\"},{\"content\":{\"connectorIds\":[\"In1\"],\"side\":\"BOTTOM\"},\"type\":\"ConnectorPlacement.EquallySpacedRectSide\",\"uuid\":\"03b25f36-aacb-41ee-af59-a85918c1221a\"}]},\"type\":\"ConnectorPlacement.EquallySpacedConnector\",\"uuid\":\"68a829ea-ceae-4477-bf03-0573732a373e\"}],\"packageUris\":[\"http://schema.mathworks.com/mf0/Connector/R2020b\"],\"version\":\"1.0\"}"
  Bus Element Out1 : Outport  PortName=VehicleSensoryFeedback
  wires:
  Bus Element In3/1 -> Brake_RR/1(Braking)
  Bus Element In4/1 -> Brake_RL/1(Braking)
  Bus Element In5/1 -> Brake_FR/1(Braking)
  Bus Element In6/1 -> Brake_FL/1(Braking)

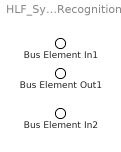
== system HLF_SystemArchitecture/Speed Limit Recognition ==
  Bus Element In1 : Inport  PortName=RGBImage
  Bus Element In2 : Inport  Port=2  PortName=EgoPosition
  Bus Element Out1 : Outport  PortName=LIN_SpeedLimit

== system HLF_SystemArchitecture/Traffic Participants Detection ==
  Bus Element In1 : Inport  PortName=RadarData
  Bus Element Out1 : Outport  PortName=CAN_confirmedTracks

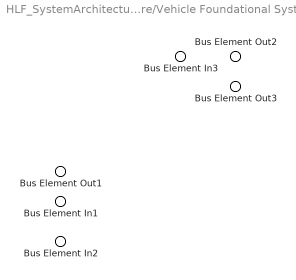
== system HLF_SystemArchitecture/Vehicle Foundational Systems ==
  Bus Element In3 : Inport  PortName=UserActions
  Bus Element In1 : Inport  Port=2  PortName=LIN_SteeringCmd
  Bus Element In2 : Inport  Port=3  PortName=LIN_Acceleration/Deceleration
  Bus Element Out3 : Outport  PortName=Braking
  Bus Element Out2 : Outport  Port=2  PortName=Acceleration
  Bus Element Out1 : Outport  Port=3  PortName=Steering

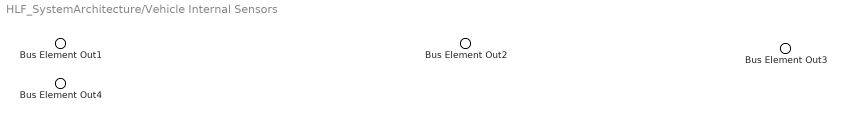
== system HLF_SystemArchitecture/Vehicle Internal Sensors ==
  Bus Element Out2 : Outport  PortName=LateralAcceleration
  Bus Element Out3 : Outport  Port=2  PortName=RollRate
  Bus Element Out1 : Outport  Port=3  PortName=YawAngleRate
  Bus Element Out4 : Outport  Port=4  PortName=LIN_LongitudinalVelocity

== system HLF_SystemArchitecture/Driver Interface/HLF Switch ==
  Bus Element Out1 : Outport  PortName=EnableHLF
  Bus Element Out2 : Outport  Port=2  PortName=DisableHLF

== system HLF_SystemArchitecture/Environment Sensors/Camera  ==
  Bus Element Out1 : Outport  PortName=RGBImage

== system HLF_SystemArchitecture/Environment Sensors/GPS Sensor ==
  Bus Element In1 : Inport  PortName=SatelliteData
  Bus Element Out1 : Outport  PortName=Pose

== system HLF_SystemArchitecture/Environment Sensors/Radar Sensor ==
  Bus Element Out1 : Outport  PortName=RadarData

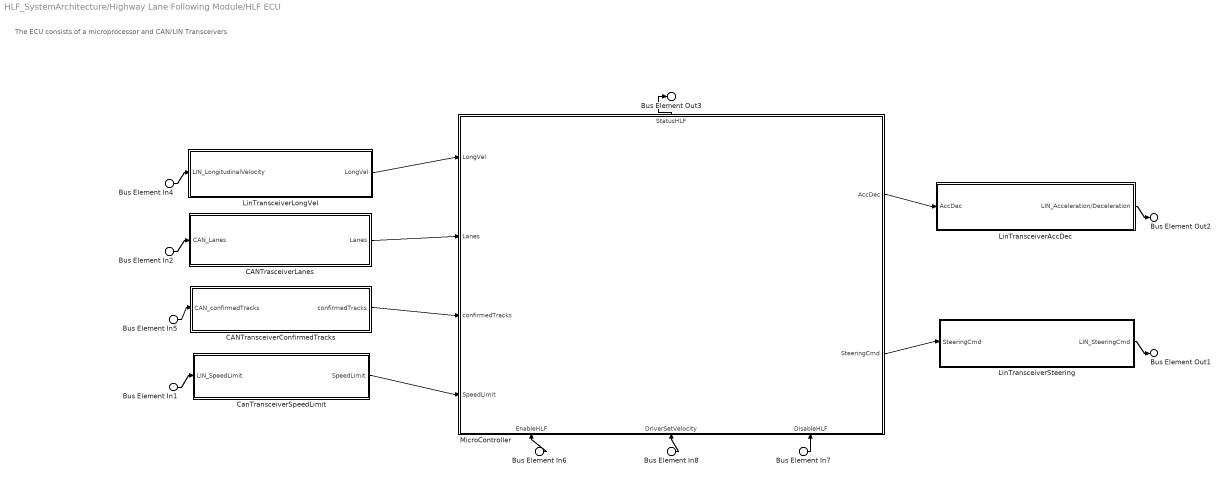
== system HLF_SystemArchitecture/Highway Lane Following Module/HLF ECU ==
  note: The ECU consists of a microprocessor and CAN/LIN Transceivers
  Bus Element In6 : Inport  PortName=EnableHLF
  Bus Element In7 : Inport  Port=2  PortName=DisableHLF
  Bus Element In8 : Inport  Port=3  PortName=DriverSetVelocity
  Bus Element In4 : Inport  Port=4  PortName=LIN_LongitudinalVelocity
  Bus Element In5 : Inport  Port=5  PortName=CAN_confirmedTracks
  Bus Element In1 : Inport  Port=6  PortName=LIN_SpeedLimit
  Bus Element In2 : Inport  Port=7  PortName=CAN_Lanes
  " MicroController" : Subsystem
      settings: PortSchema="{\"entries\":[{\"content\":{\"headerSize\":26,\"margin\":15,\"minimumSpacing\":25,\"sides\":[{\"content\":{\"connectorIds\":[\"In1\",\"In7\",\"In3\",\"In4\"]},\"type\":\"ConnectorPlacement.EquallySpacedRectSide\",\"uuid\":\"5982ae23-38c5-467f-966f-0de5138e6d7a\"},{\"content\":{\"connectorIds\":[\"Out1\",\"Out2\"],\"side\":\"RIGHT\"},\"type\":\"ConnectorPlacement.EquallySpacedRectSide\",\"uuid\":\"84362337-a9b7-4030-aff8-83ed548d578d\"},{\"content\":{\"connectorIds\":[\"Out3\"],\"side\":\"TOP\"},\"type\":\"ConnectorPlacement.EquallySpacedRectSide\",\"uuid\":\"856fe994-3ca2-486c-b816-04bdae2310a8\"},{\"content\":{\"connectorIds\":[\"In5\",\"In6\",\"In2\"],\"side\":\"BOTTOM\"},\"type\":\"ConnectorPlacement.EquallySpacedRectSide\",\"uuid\":\"3e50023d-8cdd-49e1-98f1-07624c976b94\"}]},\"type\":\"ConnectorPlacement.EquallySpacedConnector\",\"uuid\":\"ebc65c4e-e942-490a-8c6c-35e3db9f64d6\"}],\"packageUris\":[\"http://schema.mathworks.com/mf0/Connector/R2020b\"],\"version\":\"1.0\"}"
  CANTransceiverConfirmedTracks : Subsystem
      settings: PortSchema="{\"entries\":[{\"content\":{\"headerSize\":26,\"margin\":15,\"minimumSpacing\":25,\"sides\":[{\"content\":{\"connectorIds\":[\"In1\"]},\"type\":\"ConnectorPlacement.EquallySpacedRectSide\",\"uuid\":\"5982ae23-38c5-467f-966f-0de5138e6d7a\"},{\"content\":{\"connectorIds\":[\"Out1\"],\"side\":\"RIGHT\"},\"type\":\"ConnectorPlacement.EquallySpacedRectSide\",\"uuid\":\"84362337-a9b7-4030-aff8-83ed548d578d\"},{\"content\":{\"connectorIds\":[],\"side\":\"TOP\"},\"type\":\"ConnectorPlacement.EquallySpacedRectSide\",\"uuid\":\"856fe994-3ca2-486c-b816-04bdae2310a8\"}]},\"type\":\"ConnectorPlacement.EquallySpacedConnector\",\"uuid\":\"ebc65c4e-e942-490a-8c6c-35e3db9f64d6\"}],\"packageUris\":[\"http://schema.mathworks.com/mf0/Connector/R2020b\"],\"version\":\"1.0\"}"
  CANTrasceiverLanes : Subsystem
      settings: PortSchema="{\"entries\":[{\"content\":{\"headerSize\":26,\"margin\":15,\"minimumSpacing\":25,\"sides\":[{\"content\":{\"connectorIds\":[\"In1\"]},\"type\":\"ConnectorPlacement.EquallySpacedRectSide\",\"uuid\":\"5982ae23-38c5-467f-966f-0de5138e6d7a\"},{\"content\":{\"connectorIds\":[\"Out1\"],\"side\":\"RIGHT\"},\"type\":\"ConnectorPlacement.EquallySpacedRectSide\",\"uuid\":\"84362337-a9b7-4030-aff8-83ed548d578d\"},{\"content\":{\"connectorIds\":[],\"side\":\"TOP\"},\"type\":\"ConnectorPlacement.EquallySpacedRectSide\",\"uuid\":\"856fe994-3ca2-486c-b816-04bdae2310a8\"}]},\"type\":\"ConnectorPlacement.EquallySpacedConnector\",\"uuid\":\"ebc65c4e-e942-490a-8c6c-35e3db9f64d6\"}],\"packageUris\":[\"http://schema.mathworks.com/mf0/Connector/R2020b\"],\"version\":\"1.0\"}"
  CanTransceiverSpeedLimit : Subsystem
      settings: PortSchema="{\"entries\":[{\"content\":{\"headerSize\":26,\"margin\":15,\"minimumSpacing\":25,\"sides\":[{\"content\":{\"connectorIds\":[\"In1\"]},\"type\":\"ConnectorPlacement.EquallySpacedRectSide\",\"uuid\":\"5982ae23-38c5-467f-966f-0de5138e6d7a\"},{\"content\":{\"connectorIds\":[\"Out1\"],\"side\":\"RIGHT\"},\"type\":\"ConnectorPlacement.EquallySpacedRectSide\",\"uuid\":\"84362337-a9b7-4030-aff8-83ed548d578d\"},{\"content\":{\"connectorIds\":[],\"side\":\"TOP\"},\"type\":\"ConnectorPlacement.EquallySpacedRectSide\",\"uuid\":\"856fe994-3ca2-486c-b816-04bdae2310a8\"}]},\"type\":\"ConnectorPlacement.EquallySpacedConnector\",\"uuid\":\"ebc65c4e-e942-490a-8c6c-35e3db9f64d6\"}],\"packageUris\":[\"http://schema.mathworks.com/mf0/Connector/R2020b\"],\"version\":\"1.0\"}"
  LinTransceiverAccDec : Subsystem
      settings: PortSchema="{\"entries\":[{\"content\":{\"headerSize\":26,\"margin\":15,\"minimumSpacing\":25,\"sides\":[{\"content\":{\"connectorIds\":[\"In1\"]},\"type\":\"ConnectorPlacement.EquallySpacedRectSide\",\"uuid\":\"5982ae23-38c5-467f-966f-0de5138e6d7a\"},{\"content\":{\"connectorIds\":[\"Out1\"],\"side\":\"RIGHT\"},\"type\":\"ConnectorPlacement.EquallySpacedRectSide\",\"uuid\":\"84362337-a9b7-4030-aff8-83ed548d578d\"},{\"content\":{\"connectorIds\":[],\"side\":\"TOP\"},\"type\":\"ConnectorPlacement.EquallySpacedRectSide\",\"uuid\":\"856fe994-3ca2-486c-b816-04bdae2310a8\"}]},\"type\":\"ConnectorPlacement.EquallySpacedConnector\",\"uuid\":\"ebc65c4e-e942-490a-8c6c-35e3db9f64d6\"}],\"packageUris\":[\"http://schema.mathworks.com/mf0/Connector/R2020b\"],\"version\":\"1.0\"}"
  LinTransceiverLongVel : Subsystem
      settings: PortSchema="{\"entries\":[{\"content\":{\"headerSize\":26,\"margin\":15,\"minimumSpacing\":25,\"sides\":[{\"content\":{\"connectorIds\":[\"In1\"]},\"type\":\"ConnectorPlacement.EquallySpacedRectSide\",\"uuid\":\"5982ae23-38c5-467f-966f-0de5138e6d7a\"},{\"content\":{\"connectorIds\":[\"Out1\"],\"side\":\"RIGHT\"},\"type\":\"ConnectorPlacement.EquallySpacedRectSide\",\"uuid\":\"84362337-a9b7-4030-aff8-83ed548d578d\"},{\"content\":{\"connectorIds\":[],\"side\":\"TOP\"},\"type\":\"ConnectorPlacement.EquallySpacedRectSide\",\"uuid\":\"856fe994-3ca2-486c-b816-04bdae2310a8\"}]},\"type\":\"ConnectorPlacement.EquallySpacedConnector\",\"uuid\":\"ebc65c4e-e942-490a-8c6c-35e3db9f64d6\"}],\"packageUris\":[\"http://schema.mathworks.com/mf0/Connector/R2020b\"],\"version\":\"1.0\"}"
  LinTransceiverSteering : Subsystem
      settings: PortSchema="{\"entries\":[{\"content\":{\"headerSize\":26,\"margin\":15,\"minimumSpacing\":25,\"sides\":[{\"content\":{\"connectorIds\":[\"In1\"]},\"type\":\"ConnectorPlacement.EquallySpacedRectSide\",\"uuid\":\"5982ae23-38c5-467f-966f-0de5138e6d7a\"},{\"content\":{\"connectorIds\":[\"Out1\"],\"side\":\"RIGHT\"},\"type\":\"ConnectorPlacement.EquallySpacedRectSide\",\"uuid\":\"84362337-a9b7-4030-aff8-83ed548d578d\"},{\"content\":{\"connectorIds\":[],\"side\":\"TOP\"},\"type\":\"ConnectorPlacement.EquallySpacedRectSide\",\"uuid\":\"856fe994-3ca2-486c-b816-04bdae2310a8\"}]},\"type\":\"ConnectorPlacement.EquallySpacedConnector\",\"uuid\":\"ebc65c4e-e942-490a-8c6c-35e3db9f64d6\"}],\"packageUris\":[\"http://schema.mathworks.com/mf0/Connector/R2020b\"],\"version\":\"1.0\"}"
  Bus Element Out1 : Outport  PortName=LIN_SteeringCmd
  Bus Element Out2 : Outport  Port=2  PortName=LIN_Acceleration/Deceleration
  Bus Element Out3 : Outport  Port=3  PortName=StatusHLF
  wires:
  Bus Element In2/1 -> CANTrasceiverLanes/1(CAN_Lanes)
  CANTrasceiverLanes/1(Lanes) -> " MicroController"/7(Lanes)
  Bus Element In6/1 -> " MicroController"/5(EnableHLF)
  Bus Element In7/1 -> " MicroController"/2(DisableHLF)
  " MicroController"/3(StatusHLF) -> Bus Element Out3/1
  Bus Element In8/1 -> " MicroController"/6(DriverSetVelocity)
  CANTransceiverConfirmedTracks/1(confirmedTracks) -> " MicroController"/3(confirmedTracks)
  Bus Element In5/1 -> CANTransceiverConfirmedTracks/1(CAN_confirmedTracks)
  Bus Element In4/1 -> LinTransceiverLongVel/1(LIN_LongitudinalVelocity)
  LinTransceiverLongVel/1(LongVel) -> " MicroController"/1(LongVel)
  " MicroController"/1(AccDec) -> LinTransceiverAccDec/1(AccDec)
  " MicroController"/2(SteeringCmd) -> LinTransceiverSteering/1(SteeringCmd)
  LinTransceiverAccDec/1(LIN_Acceleration/Deceleration) -> Bus Element Out2/1
  LinTransceiverSteering/1(LIN_SteeringCmd) -> Bus Element Out1/1
  CanTransceiverSpeedLimit/1(SpeedLimit) -> " MicroController"/4(SpeedLimit)
  Bus Element In1/1 -> CanTransceiverSpeedLimit/1(LIN_SpeedLimit)

== system HLF_SystemArchitecture/Physical Vehicle/Brake_FL ==
  Bus Element In1 : Inport  PortName=Braking

== system HLF_SystemArchitecture/Physical Vehicle/Brake_FR ==
  Bus Element In1 : Inport  PortName=Braking

== system HLF_SystemArchitecture/Physical Vehicle/Brake_RL ==
  Bus Element In1 : Inport  PortName=Braking

== system HLF_SystemArchitecture/Physical Vehicle/Brake_RR ==
  Bus Element In1 : Inport  PortName=Braking

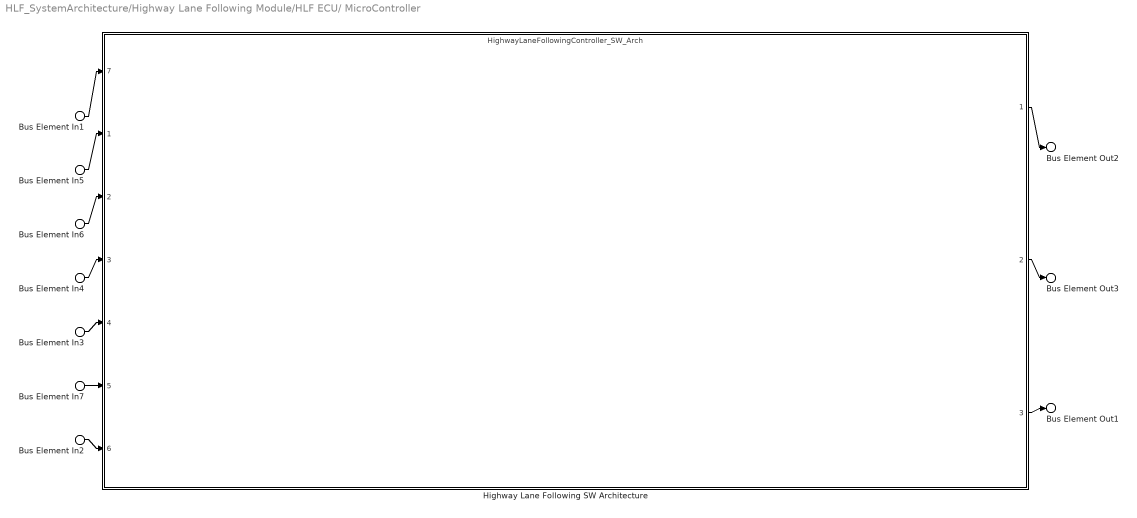
== system HLF_SystemArchitecture/Highway Lane Following Module/HLF ECU/ MicroController ==
  Bus Element In6 : Inport  PortName=LongVel
  Bus Element In3 : Inport  Port=2  PortName=DisableHLF
  Bus Element In5 : Inport  Port=3  PortName=confirmedTracks
  Bus Element In7 : Inport  Port=4  PortName=SpeedLimit
  Bus Element In2 : Inport  Port=5  PortName=EnableHLF
  Bus Element In4 : Inport  Port=6  PortName=DriverSetVelocity
  Bus Element In1 : Inport  Port=7  PortName=Lanes
  Highway Lane Following SW Architecture : ModelReference  ModelNameDialog=HighwayLaneFollowingController_SW_Arch  SimulationMode=Normal  ModelReferenceVersion=8.0
      settings: PortSchema="{\"entries\":[{\"content\":{\"headerSize\":38,\"margin\":15,\"minimumSpacing\":25,\"sides\":[{\"content\":{\"connectorIds\":[\"In7\",\"In1\",\"In2\",\"In3\",\"In4\",\"In5\",\"In6\"]},\"type\":\"ConnectorPlacement.EquallySpacedRectSide\",\"uuid\":\"a976da14-1036-413b-8707-75db1855bea5\"},{\"content\":{\"connectorIds\":[\"Out1\",\"Out2\",\"Out3\"],\"side\":\"RIGHT\"},\"type\":\"ConnectorPlacement.EquallySpacedRectSide\",\"uuid\":\"6cc185f9-955e-4f0e-a791-264a63c99544\"},{\"content\":{\"connectorIds\":[],\"side\":\"TOP\"},\"type\":\"ConnectorPlacement.EquallySpacedRectSide\",\"uuid\":\"5df0e671-9c92-4a74-a304-17df078a4265\"},{\"content\":{\"connectorIds\":[],\"side\":\"BOTTOM\"},\"type\":\"ConnectorPlacement.EquallySpacedRectSide\",\"uuid\":\"61fe1e91-c0c7-4b81-a0f1-91eab648dcce\"},{\"content\":{\"connectorIds\":[],\"side\":\"HIDDEN\"},\"type\":\"ConnectorPlacement.EquallySpacedRectSide\",\"uuid\":\"a2795b55-5f7c-44a3-8f69-8818146561ca\"}]},\"type\":\"ConnectorPlacement.EquallySpacedConnector\",\"uuid\":\"3be684c7-0fb9-41f1-bfae-e7223667cb79\"}],\"packageUris\":[\"http://schema.mathworks.com/mf0/Connector/R2020b\"],\"version\":\"1.0\"}"
  Bus Element Out2 : Outport  PortName=AccDec
  Bus Element Out3 : Outport  Port=2  PortName=SteeringCmd
  Bus Element Out1 : Outport  Port=3  PortName=StatusHLF
  wires:
  Highway Lane Following SW Architecture/1 -> Bus Element Out2/1
  Highway Lane Following SW Architecture/2 -> Bus Element Out3/1
  Highway Lane Following SW Architecture/3 -> Bus Element Out1/1
  Bus Element In6/1 -> Highway Lane Following SW Architecture/2
  Bus Element In1/1 -> Highway Lane Following SW Architecture/7
  Bus Element In5/1 -> Highway Lane Following SW Architecture/1
  Bus Element In7/1 -> Highway Lane Following SW Architecture/5
  Bus Element In2/1 -> Highway Lane Following SW Architecture/6
  Bus Element In4/1 -> Highway Lane Following SW Architecture/3
  Bus Element In3/1 -> Highway Lane Following SW Architecture/4

== system HLF_SystemArchitecture/Highway Lane Following Module/HLF ECU/CANTransceiverConfirmedTracks ==
  Bus Element In1 : Inport  PortName=CAN_confirmedTracks
  Bus Element Out1 : Outport  PortName=confirmedTracks

== system HLF_SystemArchitecture/Highway Lane Following Module/HLF ECU/CANTrasceiverLanes ==
  Bus Element In1 : Inport  PortName=CAN_Lanes
  Bus Element Out1 : Outport  PortName=Lanes

== system HLF_SystemArchitecture/Highway Lane Following Module/HLF ECU/CanTransceiverSpeedLimit ==
  Bus Element In1 : Inport  PortName=LIN_SpeedLimit
  Bus Element Out1 : Outport  PortName=SpeedLimit

== system HLF_SystemArchitecture/Highway Lane Following Module/HLF ECU/LinTransceiverAccDec ==
  Bus Element In1 : Inport  PortName=AccDec
  Bus Element Out1 : Outport  PortName=LIN_Acceleration/Deceleration

== system HLF_SystemArchitecture/Highway Lane Following Module/HLF ECU/LinTransceiverLongVel ==
  Bus Element In1 : Inport  PortName=LIN_LongitudinalVelocity
  Bus Element Out1 : Outport  PortName=LongVel

== system HLF_SystemArchitecture/Highway Lane Following Module/HLF ECU/LinTransceiverSteering ==
  Bus Element In1 : Inport  PortName=SteeringCmd
  Bus Element Out1 : Outport  PortName=LIN_SteeringCmd
